simulink model "car_model"  (R2018b)
settings: Solver=VariableStepAuto  StartTime=0.0  StopTime=10  RelTol=1e-3
undefined symbols (not defined in the file or in its folder): Ts
settings Model: Creator=Alireza  LastModifiedBy=Alireza

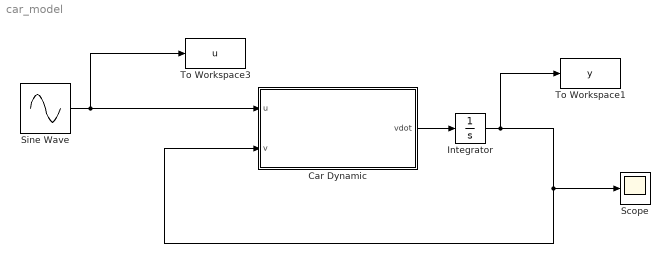
== system car_model ==
  Car Dynamic : MATLAB Function  TreatAsAtomicUnit=on
  Integrator : Integrator
  Scope : Scope
  Sine Wave : Sin  Amplitude=100  Frequency=8  SampleTime=Ts
  To Workspace1 : ToWorkspace  VariableName=y  SampleTime=Ts
      settings: Save2DSignal=2-D array (concatenate along first dimension)
  To Workspace3 : ToWorkspace  VariableName=u  SampleTime=Ts
      settings: Save2DSignal=2-D array (concatenate along first dimension)
  wires:
  Sine Wave/1 -> To Workspace3/1, Car Dynamic/1(u)
  Car Dynamic/1(vdot) -> Integrator/1
  Integrator/1 -> To Workspace1/1, Scope/1, Car Dynamic/2(v)

== matlab function car_model/Car Dynamic ==
  data: u input; vdot output; v input
function vdot = fcn(u, v)
Kc = 1;
Kf = 1;
Ka = 1;
m = 10;
vdot = (u/m)-(Kc/m)*sign(v)-(Kf/m)*v-(Ka/m)*(v^2);
